simulink model "Quadcopter_model_refined"  (R2022b)
settings: Solver=VariableStepAuto  StartTime=0.0  StopTime=10.0  RelTol=1e-3
undefined symbols (not defined in the file): Cm, Ct, g, initState, Ir, Ixx, Iyy, Izz, Length, mass
libraries: sharedtransform x4, simulink_extras x2, shared6dof x1, aerolibutil x1
settings Model: Creator=Bw Jiang  LastModifiedBy=Bw Jiang

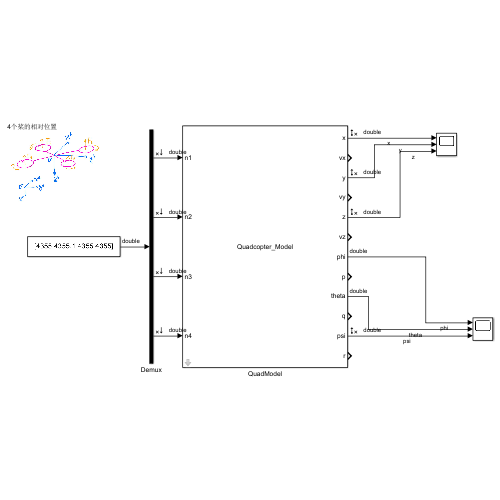
[thumbnail: Simulink's stored preview of the top-level diagram]
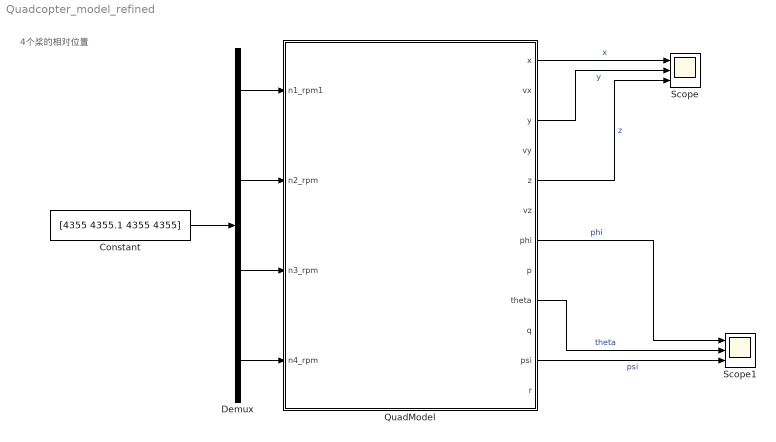
== system Quadcopter_model_refined ==
  note: 4个桨的相对位置
  Constant : Constant  Value=[4355 4355.1 4355 4355]
  Demux : Demux
  QuadModel : Subsystem  mask{g=g, mass=mass, I_xx=Ixx, I_yy=Iyy, I_zz=Izz, I_r=Ir, L=Length, C_M=Cm, C_T=Ct}
      mask prompts: g "Gravity"; I_xx "Inertia_xx"; I_yy "Inertia_yy"; I_zz "Inertia_zz"; I_r "Inertia_per_rotor"; L "Length"
      mask DialogControl ParameterGroupVar Prompt: 参数
      mask Display:
      | disp('Quadcopter_Model');
      | 
      | port_label('input', 1, 'n1');
      | port_label('input', 2, 'n2');
      | port_label('input', 3, 'n3');
      | port_label('input', 4, 'n4');
      | 
      | port_label('output', 1, 'x');
      | port_label('output', 2, 'vx');
      | port_label('output', 3, 'y');
      | port_label('output', 4, 'vy');
      | port_label('output', 5, 'z');
      | port_label('output', 6, 'vz');
      | port_label('output', 7, 'phi');
      | port_label('output', 8, 'p');
      | port_label('output', 9, 'theta');
      | port_label('output', 10, 'q');
      | port_label('output', 11, 'psi');
      | port_label('output', 12, 'r');
  Scope : Scope  NumInputPorts=3
  Scope1 : Scope  NumInputPorts=3
  wires:
  Constant/1 -> Demux/1
  Demux/4 -> QuadModel/4(n4_rpm)
  Demux/1 -> QuadModel/1(n1_rpm1)
  Demux/3 -> QuadModel/3(n3_rpm)
  Demux/2 -> QuadModel/2(n2_rpm)
  QuadModel/1(x) -> Scope/1  "x"
  QuadModel/3(y) -> Scope/2  "y"
  QuadModel/5(z) -> Scope/3  "z"
  QuadModel/11(psi) -> Scope1/3  "psi"
  QuadModel/7(phi) -> Scope1/1  "phi"
  QuadModel/9(theta) -> Scope1/2  "theta"

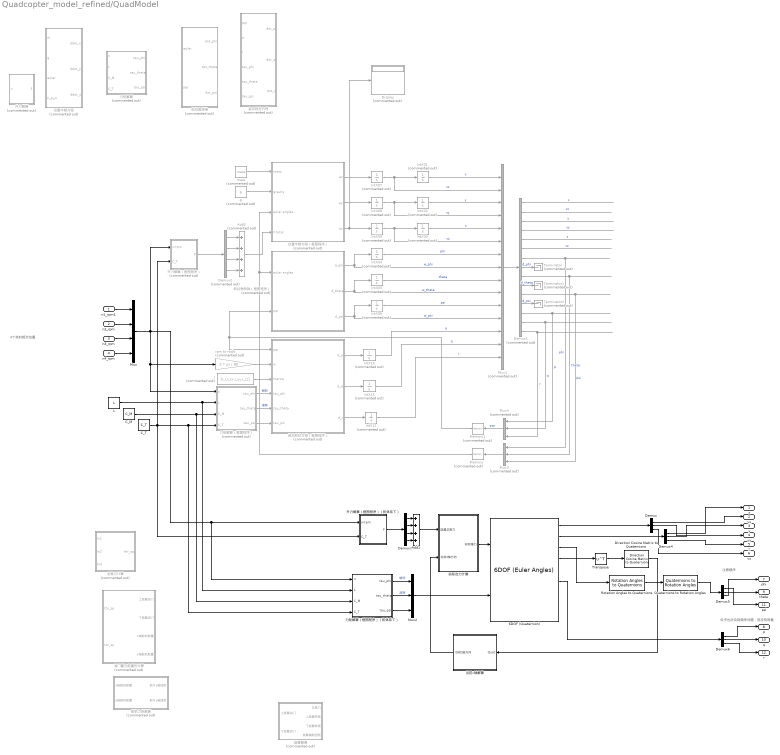
== system Quadcopter_model_refined/QuadModel ==
  note: 似乎也涉及到顺序问题，但没有用着
  note: 注意顺序
  note: 4个桨的相对位置
  n1_rpm1 : Inport
  n2_rpm : Inport  Port=2
  n3_rpm : Inport  Port=3
  n4_rpm : Inport  Port=4
  6DOF (Quaternion) : shared6dof/6DOF (Euler Angles)  units=Metric (MKS)  mtype=Fixed  rep=Euler Angles  xme_0=[initState.x, initState.y, initState.z]  Vm_0=[initState.vx, initState.vy, initState.vz]  eul_0=[initState.phi, initState.theta, initState.psi]  pm_0=[initState.p, initState.q, initState.r]  mass_0=mass  mass_e=0.5  mass_f=2.0  inertia=[Ixx, 0, 0; 0, Iyy, 0; 0, 0, Izz]  inertia_e=eye(3)  inertia_f=2*eye(3)  k_quat=Vehicle.SixDOF.quatGain  vre_flag=on  abi_flag=on  aMode=aMode  xme_statename=''  Vm_statename=''  eul_statename=''  quat_statename=''  pm_statename=''  mass_statename=''
  Add1 : Sum  Inputs=++++
  Add2 : Sum  Commented=on  Inputs=++++
  C_M : Constant  Value=C_M
  C_T : Constant  Value=C_T
  Demux{,4..6} (4 alike) : Demux  Outputs=3
  Demux1 : Demux  Commented=on  Outputs=15
  Demux2 : Demux  Commented=on
  Demux3 : Demux
  Direction Cosine Matrix to Quaternions : sharedtransform/Direction Cosine Matrix  to Quaternions  aMode=0  action=None  tolerance=eps(2)
  Display : Display  Commented=on
  I : Constant  Commented=on  Value=[I_r,I_xx,I_yy,I_zz]
  IntX01 : Integrator  Commented=on
  IntX02 : Integrator  Commented=on
  IntX03 : Integrator  Commented=on
  IntX04 : Integrator  Commented=on
  IntX05 : Integrator  Commented=on
  IntX06 : Integrator  Commented=on
  IntX07 : Integrator  Commented=on
  IntX08 : Integrator  Commented=on
  IntX09 : Integrator  Commented=on
  IntX10 : Integrator  Commented=on
  IntX11 : Integrator  Commented=on
  IntX12 : Integrator  Commented=on
  L : Constant  Value=L
  Memory : Memory  Commented=on  InheritSampleTime=on
  Memory1 : Memory  Commented=on  InheritSampleTime=on
  Mux : Mux
  Mux1 : Mux  Commented=on  Inputs=15
  Mux2 : Mux  Inputs=3
  Mux3 : Mux  Commented=on  Inputs=3
  Mux4 : Mux  Commented=on  Inputs=3
  Quaternions to Rotation Angles : sharedtransform/Quaternions to Rotation Angles  rotationOrder=XYZ  aMode=aMode
  Rotation Angles to Quaternions : sharedtransform/Rotation Angles to Quaternions  rotationOrder=ZYX  aMode=aMode
  Terminator : Terminator  Commented=on
  Terminator1 : Terminator  Commented=on
  Terminator2 : Terminator  Commented=on
  Transpose : Math  Operator=transpose
  g : Constant  Commented=on  Value=g
  mass : Constant  Commented=on  Value=mass
  rpm to rad/s : Gain  Commented=on  Gain=2 * pi / 60
  位置牛顿方程 : MATLAB Function  Commented=on  TreatAsAtomicUnit=on
  位置牛顿方程（框图程序） : Subsystem  Commented=on
  力矩解算 : MATLAB Function  Commented=on  TreatAsAtomicUnit=on
  力矩解算（框图程序） : Subsystem  Commented=on
  力矩解算（框图程序）（机体系下） : Subsystem
  升力解算 : MATLAB Function  Commented=on  TreatAsAtomicUnit=on
  升力解算（框图程序） : Subsystem  Commented=on
  升力解算（框图程序）（机体系下） : Subsystem
  姿态欧拉方程 : MATLAB Function  Commented=on  TreatAsAtomicUnit=on
  姿态欧拉方程（框图程序） : Subsystem  Commented=on
  实际合力计算 : Subsystem
  当前z轴解算 : Subsystem
  总推力计算 : Subsystem  Commented=on
  旋翼解算 : Subsystem  Commented=on
  欧拉角转换 : MATLAB Function  Commented=on  TreatAsAtomicUnit=on
  欧拉角转换（框图程序） : Subsystem  Commented=on
  油门量与舵量的计算 : Subsystem  Commented=on
  舵机力矩解算 : Subsystem  Commented=on
  x : Outport
  vx : Outport  Port=2
  y : Outport  Port=3
  vy : Outport  Port=4
  z : Outport  Port=5
  vz : Outport  Port=6
  phi : Outport  Port=7
  p : Outport  Port=8
  theta : Outport  Port=9
  q : Outport  Port=10
  psi : Outport  Port=11
  r : Outport  Port=12
  wires:
  Demux1/15 -> Mux4/3  "r"
  Demux1/13 -> Mux4/1  "p"
  Mux4/1 -> Memory1/1  "pqr"
  Demux1/9 -> Mux3/2  "theta"
  Demux1/1 -> ?  "x"
  Demux1/2 -> ?  "vx"
  Demux1/11 -> Mux3/3  "psi"
  Demux1/4 -> ?  "vy"
  Demux1/3 -> ?  "y"
  Demux1/5 -> ?  "z"
  Mux1/1 -> Demux1/1
  Demux1/6 -> ?  "vz"
  Demux1/7 -> Mux3/1  "phi"
  Mux3/1 -> Memory/1
  Demux1/14 -> Mux4/2  "q"
  Demux1/8 -> Terminator/1  "d_phi"
  Demux1/10 -> Terminator1/1  "d_theta"
  Demux1/12 -> Terminator2/1  "d_psi"
  n1_rpm1/1 -> Mux/1
  n2_rpm/1 -> Mux/2
  n4_rpm/1 -> Mux/4
  n3_rpm/1 -> Mux/3
  欧拉角转换（框图程序）/2(d_theta) -> IntX05/1, Mux1/10  "w_theta"
  欧拉角转换（框图程序）/3(d_psi) -> IntX06/1, Mux1/12  "w_psi"
  欧拉角转换（框图程序）/1(d_phi) -> IntX04/1, Mux1/8  "w_phi"
  力矩解算（框图程序）/3(tau_psi) -> 姿态欧拉方程（框图程序）/6(tau_psi)
  力矩解算（框图程序）/2(tau_theta) -> 姿态欧拉方程（框图程序）/5(tau_theta)  "滚转"
  姿态欧拉方程（框图程序）/2(d_q) -> IntX11/1
  姿态欧拉方程（框图程序）/3(d_r) -> IntX12/1
  mass/1 -> 位置牛顿方程（框图程序）/1(mass)
  Add2/1 -> 位置牛顿方程（框图程序）/4(F total)
  g/1 -> 位置牛顿方程（框图程序）/2(gravity)
  位置牛顿方程（框图程序）/3(az) -> Display/1, IntX09/1
  位置牛顿方程（框图程序）/2(ay) -> IntX08/1
  IntX05/1 -> Mux1/9  "theta"
  力矩解算（框图程序）/1(tau_phi) -> 姿态欧拉方程（框图程序）/4(tau_phi)  "俯仰"
  IntX07/1 -> IntX01/1, Mux1/2  "vx"
  IntX02/1 -> Mux1/3  "y"
  Demux2/3 -> Add2/3
  IntX12/1 -> Mux1/15  "r"
  rpm to rad/s/1 -> 姿态欧拉方程（框图程序）/2(w)
  IntX06/1 -> Mux1/11  "psi"
  IntX08/1 -> Mux1/4, IntX02/1  "vy"
  Mux/1 -> 力矩解算（框图程序）（机体系下）/1(n), 升力解算（框图程序）（机体系下）/1(n/rpm), 力矩解算（框图程序）/1(n), rpm to rad/s/1, 升力解算（框图程序）/1(n/rpm)
  Memory1/1 -> 欧拉角转换（框图程序）/2(pqr), 姿态欧拉方程（框图程序）/1(pqr)
  位置牛顿方程（框图程序）/1(ax) -> IntX07/1
  Demux2/1 -> Add2/1
  IntX01/1 -> Mux1/1  "x"
  IntX11/1 -> Mux1/14  "q"
  姿态欧拉方程（框图程序）/1(d_p) -> IntX10/1
  IntX04/1 -> Mux1/7  "phi"
  Demux2/2 -> Add2/2
  L/1 -> 力矩解算（框图程序）（机体系下）/2(L), 力矩解算（框图程序）/2(L)
  I/1 -> 姿态欧拉方程（框图程序）/3(Inertia)
  C_M/1 -> 力矩解算（框图程序）（机体系下）/3(C_M), 力矩解算（框图程序）/3(C_M)
  升力解算（框图程序）/1(F) -> Demux2/1
  C_T/1 -> 升力解算（框图程序）（机体系下）/2(C_T), 升力解算（框图程序）/2(C_T), 力矩解算（框图程序）（机体系下）/4(C_T), 力矩解算（框图程序）/4(C_T)
  IntX03/1 -> Mux1/5  "z"
  Demux2/4 -> Add2/4
  IntX09/1 -> Mux1/6, IntX03/1  "vz"
  IntX10/1 -> Mux1/13  "p"
  Memory/1 -> 位置牛顿方程（框图程序）/3(eular angles), 欧拉角转换（框图程序）/1(eular angles)
  实际合力计算/1(实际推力) -> 6DOF (Quaternion)/1
  6DOF (Quaternion)/4 -> Transpose/1
  Transpose/1 -> Direction Cosine Matrix to Quaternions/1
  Direction Cosine Matrix to Quaternions/1 -> 当前z轴解算/1(Quat)
  当前z轴解算/1(当前z轴方向) -> 实际合力计算/2(当前z轴方向)
  Demux3/1 -> Add1/1
  Demux3/4 -> Add1/4
  升力解算（框图程序）（机体系下）/1(F) -> Demux3/1
  Demux3/2 -> Add1/2
  Demux3/3 -> Add1/3
  Add1/1 -> 实际合力计算/1(旋翼总推力)
  力矩解算（框图程序）（机体系下）/3(tau_psi) -> Mux2/3
  力矩解算（框图程序）（机体系下）/2(tau_theta) -> Mux2/2  "滚转"
  力矩解算（框图程序）（机体系下）/1(tau_phi) -> Mux2/1  "俯仰"
  Mux2/1 -> 6DOF (Quaternion)/2
  6DOF (Quaternion)/1 -> Demux/1
  6DOF (Quaternion)/2 -> Demux4/1
  Demux4/1 -> x/1
  Demux4/2 -> y/1
  Demux4/3 -> z/1
  Demux/1 -> vx/1
  Demux/2 -> vy/1
  Demux/3 -> vz/1
  6DOF (Quaternion)/3 -> Rotation Angles to Quaternions/1
  Rotation Angles to Quaternions/1 -> Quaternions to Rotation Angles/1
  Quaternions to Rotation Angles/1 -> Demux5/1
  Demux5/1 -> psi/1
  Demux5/2 -> theta/1
  Demux5/3 -> phi/1
  6DOF (Quaternion)/6 -> Demux6/1
  Demux6/1 -> p/1
  Demux6/2 -> q/1
  Demux6/3 -> r/1

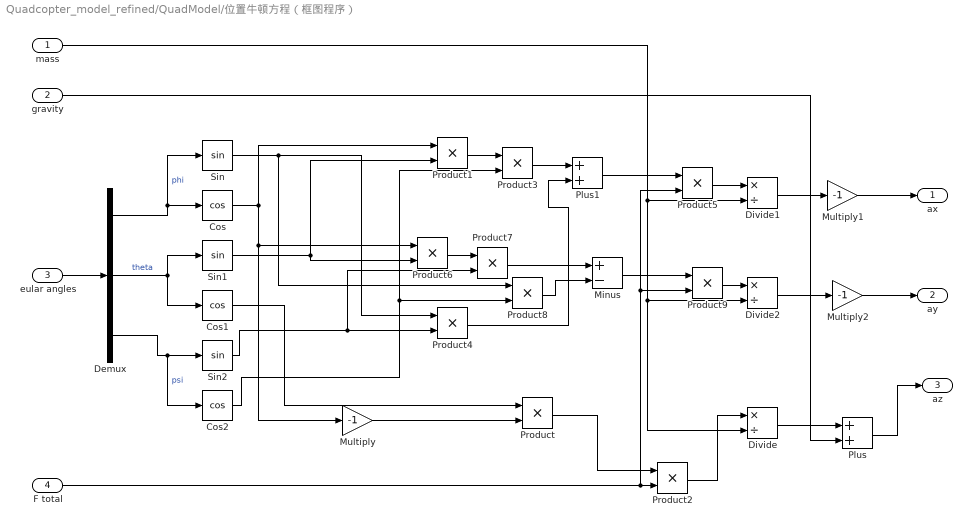
== system Quadcopter_model_refined/QuadModel/位置牛顿方程（框图程序） ==
  mass : Inport
  gravity : Inport  Port=2
  eular angles : Inport  Port=3
  F total : Inport  Port=4
  Cos : Trigonometry  Operator=cos
  Cos1 : Trigonometry  Operator=cos
  Cos2 : Trigonometry  Operator=cos
  Demux : Demux  Outputs=3
  Divide : Product  Inputs=*/
  Divide1 : Product  Inputs=*/
  Divide2 : Product  Inputs=*/
  Minus : Sum  Inputs=+-
  Multiply : Gain  Gain=-1
  Multiply1 : Gain  Gain=-1
  Multiply2 : Gain  Gain=-1
  Plus : Sum
  Plus1 : Sum
  Product{,1..9} (10 alike) : Product
  Sin : Trigonometry
  Sin1 : Trigonometry
  Sin2 : Trigonometry
  ax : Outport
  ay : Outport  Port=2
  az : Outport  Port=3
  wires:
  eular angles/1 -> Demux/1
  Demux/1 -> Sin/1, Cos/1  "phi"
  Demux/2 -> Sin1/1, Cos1/1  "theta"
  Demux/3 -> Cos2/1, Sin2/1  "psi"
  Cos/1 -> Product6/1, Multiply/1, Product1/1
  Multiply/1 -> Product/2
  Cos1/1 -> Product/1
  F total/1 -> Product5/2, Product9/2, Product2/2
  Product/1 -> Product2/1
  Product2/1 -> Divide/1
  mass/1 -> Divide2/2, Divide/2, Divide1/2
  Divide/1 -> Plus/1
  gravity/1 -> Plus/2
  Plus/1 -> az/1
  Sin1/1 -> Product1/2, Product6/2
  Product1/1 -> Product3/1
  Cos2/1 -> Product8/2, Product3/2
  Product3/1 -> Plus1/1
  Sin/1 -> Product8/1, Product4/1
  Sin2/1 -> Product7/2, Product4/2
  Product4/1 -> Plus1/2
  Plus1/1 -> Product5/1
  Product5/1 -> Divide1/1
  Divide1/1 -> Multiply1/1
  Multiply1/1 -> ax/1
  Product6/1 -> Product7/1
  Product7/1 -> Minus/1
  Product8/1 -> Minus/2
  Minus/1 -> Product9/1
  Product9/1 -> Divide2/1
  Multiply2/1 -> ay/1
  Divide2/1 -> Multiply2/1

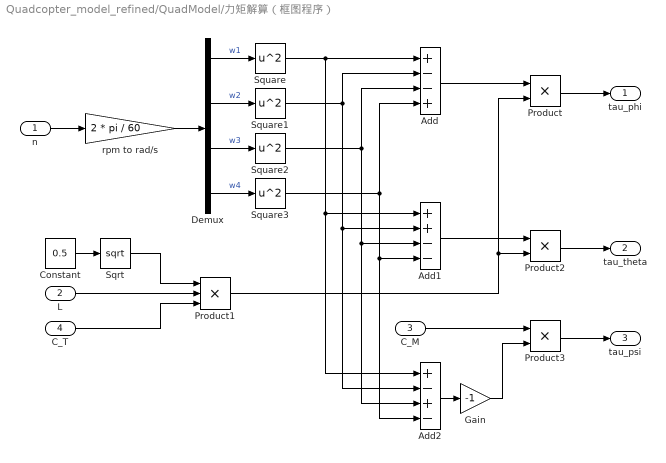
== system Quadcopter_model_refined/QuadModel/力矩解算（框图程序） ==
  n : Inport
  L : Inport  Port=2
  C_M : Inport  Port=3
  C_T : Inport  Port=4
  Add : Sum  Inputs=+--+
  Add1 : Sum  Inputs=++--
  Add2 : Sum  Inputs=+-+-
  Constant : Constant  Value=0.5
  Demux : Demux
  Gain : Gain  Gain=-1
  Product : Product
  Product1 : Product  Inputs=3
  Product2 : Product
  Product3 : Product
  Sqrt : Sqrt
  Square{,1..3} (4 alike) : Math  Operator=square
  rpm to rad/s : Gain  Gain=2 * pi / 60
  tau_phi : Outport
  tau_theta : Outport  Port=2
  tau_psi : Outport  Port=3
  wires:
  rpm to rad/s/1 -> Demux/1
  n/1 -> rpm to rad/s/1
  Demux/1 -> Square/1  "w1"
  Demux/2 -> Square1/1  "w2"
  Demux/3 -> Square2/1  "w3"
  Demux/4 -> Square3/1  "w4"
  Square/1 -> Add1/1, Add2/1, Add/1
  Square1/1 -> Add1/2, Add2/2, Add/2
  Square2/1 -> Add2/3, Add1/3, Add/3
  Square3/1 -> Add2/4, Add1/4, Add/4
  Add/1 -> Product/1
  L/1 -> Product1/2
  C_T/1 -> Product1/3
  Constant/1 -> Sqrt/1
  Sqrt/1 -> Product1/1
  Product1/1 -> Product/2, Product2/2
  Product/1 -> tau_phi/1
  Add1/1 -> Product2/1
  Product2/1 -> tau_theta/1
  Add2/1 -> Gain/1
  C_M/1 -> Product3/1
  Product3/1 -> tau_psi/1
  Gain/1 -> Product3/2

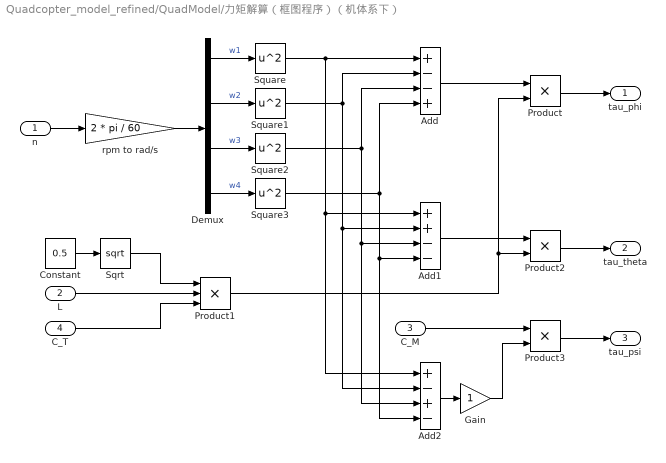
== system Quadcopter_model_refined/QuadModel/力矩解算（框图程序）（机体系下） ==
  n : Inport
  L : Inport  Port=2
  C_M : Inport  Port=3
  C_T : Inport  Port=4
  Add : Sum  Inputs=+--+
  Add1 : Sum  Inputs=++--
  Add2 : Sum  Inputs=+-+-
  Constant : Constant  Value=0.5
  Demux : Demux
  Gain : Gain
  Product : Product
  Product1 : Product  Inputs=3
  Product2 : Product
  Product3 : Product
  Sqrt : Sqrt
  Square{,1..3} (4 alike) : Math  Operator=square
  rpm to rad/s : Gain  Gain=2 * pi / 60
  tau_phi : Outport
  tau_theta : Outport  Port=2
  tau_psi : Outport  Port=3
  wires:
  rpm to rad/s/1 -> Demux/1
  n/1 -> rpm to rad/s/1
  Demux/1 -> Square/1  "w1"
  Demux/2 -> Square1/1  "w2"
  Demux/3 -> Square2/1  "w3"
  Demux/4 -> Square3/1  "w4"
  Square/1 -> Add1/1, Add2/1, Add/1
  Square1/1 -> Add1/2, Add2/2, Add/2
  Square2/1 -> Add2/3, Add1/3, Add/3
  Square3/1 -> Add2/4, Add1/4, Add/4
  Add/1 -> Product/1
  L/1 -> Product1/2
  C_T/1 -> Product1/3
  Constant/1 -> Sqrt/1
  Sqrt/1 -> Product1/1
  Product1/1 -> Product/2, Product2/2
  Product/1 -> tau_phi/1
  Add1/1 -> Product2/1
  Product2/1 -> tau_theta/1
  Add2/1 -> Gain/1
  C_M/1 -> Product3/1
  Product3/1 -> tau_psi/1
  Gain/1 -> Product3/2

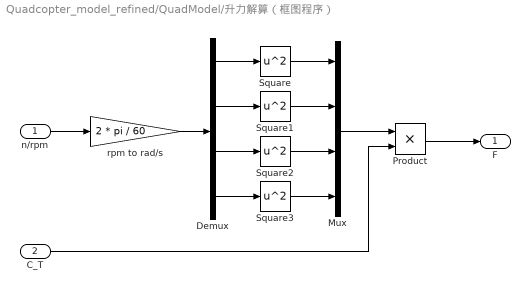
== system Quadcopter_model_refined/QuadModel/升力解算（框图程序） ==
  n/rpm : Inport
  C_T : Inport  Port=2
  Demux : Demux
  Mux : Mux
  Product : Product
  Square{,1..3} (4 alike) : Math  Operator=square
  rpm to rad/s : Gain  Gain=2 * pi / 60
  F : Outport
  wires:
  n/rpm/1 -> rpm to rad/s/1
  rpm to rad/s/1 -> Demux/1
  Demux/1 -> Square/1
  Demux/2 -> Square1/1
  Demux/3 -> Square2/1
  Demux/4 -> Square3/1
  Square3/1 -> Mux/4
  Square2/1 -> Mux/3
  Square1/1 -> Mux/2
  Square/1 -> Mux/1
  Mux/1 -> Product/1
  C_T/1 -> Product/2
  Product/1 -> F/1

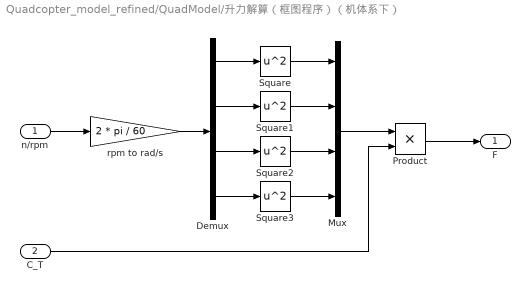
== system Quadcopter_model_refined/QuadModel/升力解算（框图程序）（机体系下） ==
  n/rpm : Inport
  C_T : Inport  Port=2
  Demux : Demux
  Mux : Mux
  Product : Product
  Square{,1..3} (4 alike) : Math  Operator=square
  rpm to rad/s : Gain  Gain=2 * pi / 60
  F : Outport
  wires:
  n/rpm/1 -> rpm to rad/s/1
  rpm to rad/s/1 -> Demux/1
  Demux/1 -> Square/1
  Demux/2 -> Square1/1
  Demux/3 -> Square2/1
  Demux/4 -> Square3/1
  Square3/1 -> Mux/4
  Square2/1 -> Mux/3
  Square1/1 -> Mux/2
  Square/1 -> Mux/1
  Mux/1 -> Product/1
  C_T/1 -> Product/2
  Product/1 -> F/1

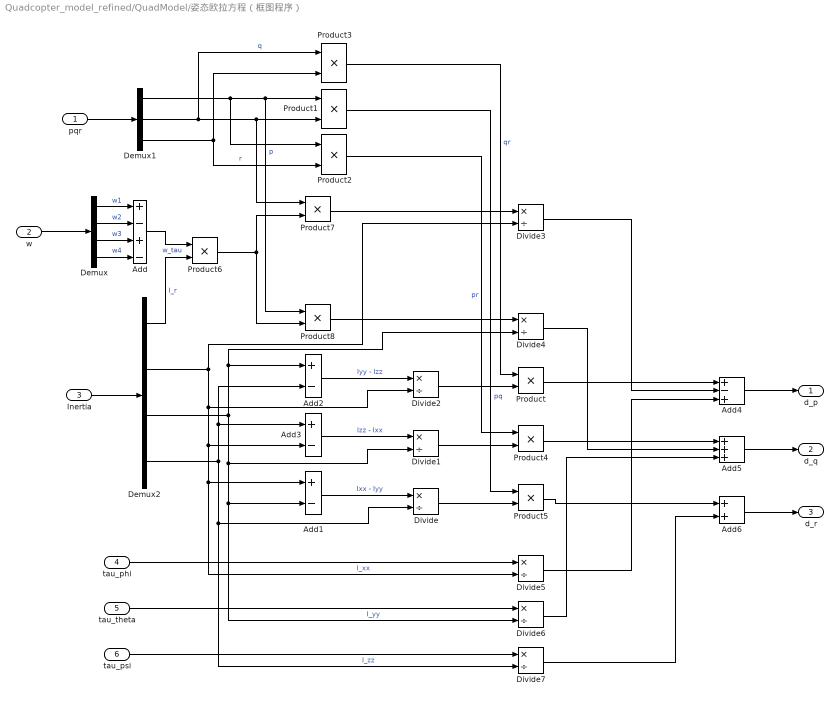
== system Quadcopter_model_refined/QuadModel/姿态欧拉方程（框图程序） ==
  pqr : Inport
  w : Inport  Port=2
  Inertia : Inport  Port=3
  tau_phi : Inport  Port=4
  tau_theta : Inport  Port=5
  tau_psi : Inport  Port=6
  Add : Sum  Inputs=+-+-
  Add1 : Sum  Inputs=+-
  Add2 : Sum  Inputs=+-
  Add3 : Sum  Inputs=+-
  Add4 : Sum  Inputs=+-+
  Add5 : Sum  Inputs=+++
  Add6 : Sum
  Demux : Demux
  Demux1 : Demux  Outputs=3
  Demux2 : Demux
  Divide{,1..7} (8 alike) : Product  Inputs=*/
  Product{,1..8} (9 alike) : Product
  d_p : Outport
  d_q : Outport  Port=2
  d_r : Outport  Port=3
  wires:
  w/1 -> Demux/1
  pqr/1 -> Demux1/1
  Inertia/1 -> Demux2/1
  Demux/1 -> Add/1  "w1"
  Demux/2 -> Add/2  "w2"
  Demux/3 -> Add/3  "w3"
  Demux/4 -> Add/4  "w4"
  Demux2/2 -> Add3/2, Add1/1, Divide5/2, Divide2/2, Divide3/2  "I_xx"
  Demux2/3 -> Divide4/2, Add2/1, Divide1/2, Divide6/2, Add1/2  "I_yy"
  Demux2/4 -> Add2/2, Add3/1, Divide7/2, Divide/2  "I_zz"
  Add1/1 -> Divide/1  "Ixx - Iyy"
  Add3/1 -> Divide1/1  "Izz - Ixx"
  Add2/1 -> Divide2/1  "Iyy - Izz"
  Divide2/1 -> Product/2
  Demux1/2 -> Product3/1, Product1/2, Product7/1  "q"
  Demux1/1 -> Product2/1, Product1/1, Product8/1  "p"
  Demux1/3 -> Product2/2, Product3/2  "r"
  Divide/1 -> Product5/2
  Divide1/1 -> Product4/2
  Product3/1 -> Product/1  "qr"
  Product1/1 -> Product5/1  "pq"
  Product2/1 -> Product4/1  "pr"
  Add/1 -> Product6/1  "w_tau"
  Demux2/1 -> Product6/2  "I_r"
  Product6/1 -> Product8/2, Product7/2
  Product7/1 -> Divide3/1
  Product8/1 -> Divide4/1
  tau_phi/1 -> Divide5/1
  tau_theta/1 -> Divide6/1
  tau_psi/1 -> Divide7/1
  Product/1 -> Add4/1
  Divide3/1 -> Add4/2
  Divide5/1 -> Add4/3
  Product4/1 -> Add5/1
  Divide4/1 -> Add5/2
  Divide6/1 -> Add5/3
  Add4/1 -> d_p/1
  Add5/1 -> d_q/1
  Product5/1 -> Add6/1
  Divide7/1 -> Add6/2
  Add6/1 -> d_r/1

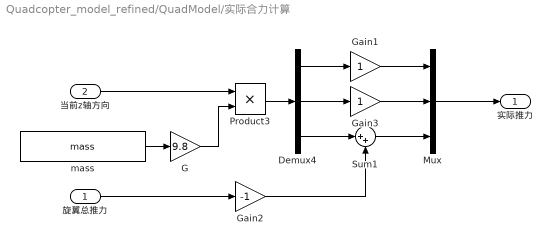
== system Quadcopter_model_refined/QuadModel/实际合力计算 ==
  旋翼总推力 : Inport
  当前z轴方向 : Inport  Port=2
  Demux4 : Demux  Outputs=3
  G : Gain  Gain=9.8
  Gain1 : Gain
  Gain2 : Gain  Gain=-1
  Gain3 : Gain
  Mux : Mux  Inputs=3
  Product3 : Product
  Sum1 : Sum  Inputs=|++
  mass : Constant  Value=mass
  实际推力 : Outport
  wires:
  Demux4/1 -> Gain1/1
  当前z轴方向/1 -> Product3/1
  G/1 -> Product3/2
  Sum1/1 -> Mux/3
  Demux4/2 -> Gain3/1
  mass/1 -> G/1
  Product3/1 -> Demux4/1
  Mux/1 -> 实际推力/1
  旋翼总推力/1 -> Gain2/1
  Gain1/1 -> Mux/1
  Gain3/1 -> Mux/2
  Demux4/3 -> Sum1/1
  Gain2/1 -> Sum1/2

== system Quadcopter_model_refined/QuadModel/当前z轴解算 ==
  Quat : Inport
  Demux5 : Demux  Outputs=3
  Display : Display
  Display1 : Display
  Quaternion Inverse : aerolibutil/Quaternion Inverse
  Quaternions to Direction Cosine Matrix : sharedtransform/Quaternions to  Direction Cosine Matrix  aMode=aMode
  Reshape2 : Reshape  OutputDimensionality=Row vector (2-D)
  ez : Scope
  一列一列地读取形成向量 : Reshape  OutputDimensionality=Column vector (2-D)
  当前z轴方向 : Outport
  wires:
  Quat/1 -> Quaternion Inverse/1
  Demux5/3 -> Reshape2/1
  Reshape2/1 -> 当前z轴方向/1, ez/1
  Quaternions to Direction Cosine Matrix/1 -> Display/1, 一列一列地读取形成向量/1
  一列一列地读取形成向量/1 -> Display1/1, Demux5/1
  Quaternion Inverse/1 -> Quaternions to Direction Cosine Matrix/1

== system Quadcopter_model_refined/QuadModel/总推力计算 ==
  In1 : Inport
  In2 : Inport  Port=2
  In3 : Inport  Port=3
  Sqrt : Sqrt
  Square : Math  Operator=square
  Square1 : Math  Operator=square
  Square2 : Math  Operator=square
  Sum1 : Sum  Inputs=+++
  thr_sp : Outport
  wires:
  Sum1/1 -> Sqrt/1
  Square1/1 -> Sum1/2
  Square/1 -> Sum1/1
  Square2/1 -> Sum1/3
  Sqrt/1 -> thr_sp/1  "thr_sp"
  In2/1 -> Square1/1
  In3/1 -> Square2/1
  In1/1 -> Square/1

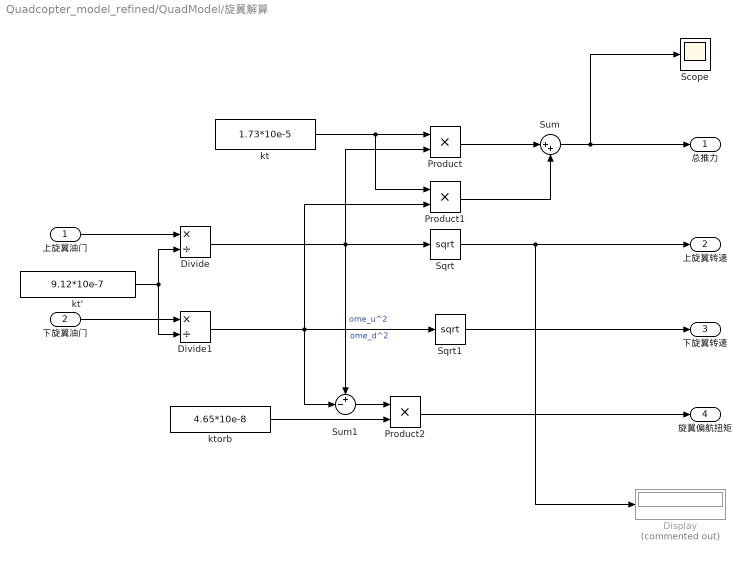
== system Quadcopter_model_refined/QuadModel/旋翼解算 ==
  上旋翼油门 : Inport
  下旋翼油门 : Inport  Port=2
  Display : Display  Commented=on
  Divide : Product  Inputs=*/
  Divide1 : Product  Inputs=*/
  Product : Product
  Product1 : Product
  Product2 : Product
  Scope : Scope
  Sqrt : Sqrt
  Sqrt1 : Sqrt
  Sum : Sum  Inputs=|++
  Sum1 : Sum  Inputs=+-|
  kt : Constant  Value=1.73*10e-5
  kt' : Constant  Value=9.12*10e-7
  ktorb : Constant  Value=4.65*10e-8
  总推力 : Outport
  上旋翼转速 : Outport  Port=2
  下旋翼转速 : Outport  Port=3
  旋翼偏航扭矩 : Outport  Port=4
  wires:
  上旋翼油门/1 -> Divide/1
  kt'/1 -> Divide1/2, Divide/2
  下旋翼油门/1 -> Divide1/1
  Divide/1 -> Sqrt/1, Product/2, Sum1/1  "ome_u^2"
  Sqrt/1 -> Display/1, 上旋翼转速/1
  Divide1/1 -> Sqrt1/1, Product1/2, Sum1/2  "ome_d^2"
  Sqrt1/1 -> 下旋翼转速/1
  kt/1 -> Product/1, Product1/1
  Product/1 -> Sum/1
  Sum/1 -> Scope/1, 总推力/1
  Product1/1 -> Sum/2
  Sum1/1 -> Product2/1
  ktorb/1 -> Product2/2
  Product2/1 -> 旋翼偏航扭矩/1

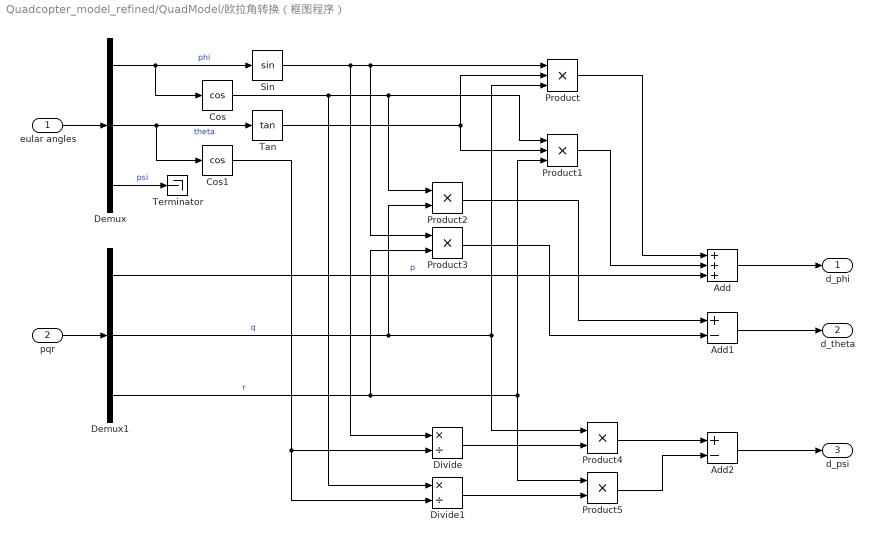
== system Quadcopter_model_refined/QuadModel/欧拉角转换（框图程序） ==
  eular angles : Inport
  pqr : Inport  Port=2
  Add : Sum  Inputs=+++
  Add1 : Sum  Inputs=+-
  Add2 : Sum  Inputs=+-
  Cos : Trigonometry  Operator=cos
  Cos1 : Trigonometry  Operator=cos
  Demux : Demux  Outputs=3
  Demux1 : Demux  Outputs=3
  Divide : Product  Inputs=*/
  Divide1 : Product  Inputs=*/
  Product : Product  Inputs=3
  Product1 : Product  Inputs=3
  Product{2..5} (4 alike) : Product
  Sin : Trigonometry
  Tan : Trigonometry  Operator=tan
  Terminator : Terminator
  d_phi : Outport
  d_theta : Outport  Port=2
  d_psi : Outport  Port=3
  wires:
  eular angles/1 -> Demux/1
  pqr/1 -> Demux1/1
  Demux1/1 -> Add/3  "p"
  Add/1 -> d_phi/1
  Add1/1 -> d_theta/1
  Add2/1 -> d_psi/1
  Demux/1 -> Sin/1, Cos/1  "phi"
  Demux/2 -> Cos1/1, Tan/1  "theta"
  Demux/3 -> Terminator/1  "psi"
  Demux1/2 -> Product2/2, Product4/1, Product/3  "q"
  Sin/1 -> Divide/1, Product3/1, Product/1
  Tan/1 -> Product1/2, Product/2
  Cos/1 -> Divide1/1, Product2/1, Product1/1
  Demux1/3 -> Product3/2, Product1/3, Product5/1  "r"
  Product/1 -> Add/1
  Product1/1 -> Add/2
  Product2/1 -> Add1/1
  Product3/1 -> Add1/2
  Cos1/1 -> Divide1/2, Divide/2
  Divide/1 -> Product4/2
  Product4/1 -> Add2/1
  Divide1/1 -> Product5/2
  Product5/1 -> Add2/2

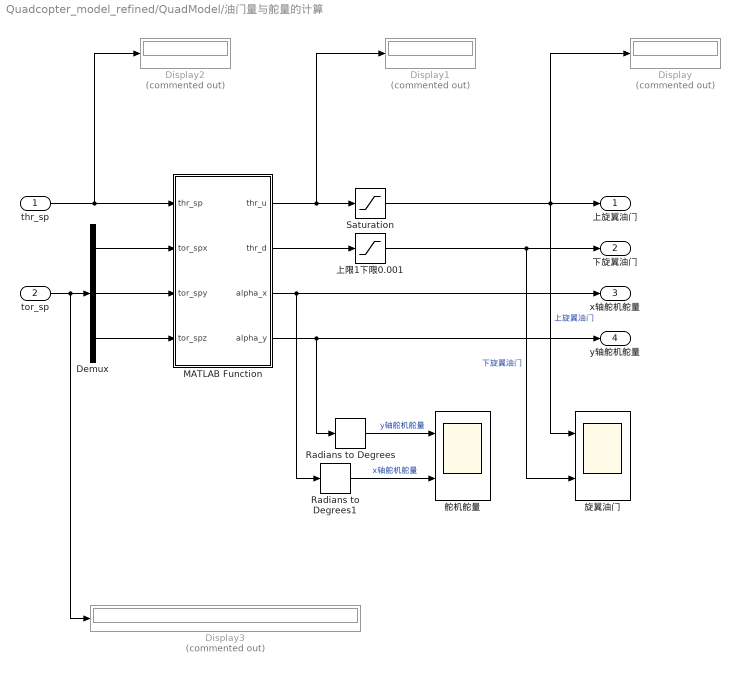
== system Quadcopter_model_refined/QuadModel/油门量与舵量的计算 ==
  thr_sp : Inport
  tor_sp : Inport  Port=2
  Demux : Demux  Outputs=3
  Display{,1..3} (4 alike) : Display  Commented=on
  MATLAB Function : MATLAB Function  TreatAsAtomicUnit=on
  Radians to Degrees : simulink_extras/Transformations/Radians to Degrees
  Radians to Degrees1 : simulink_extras/Transformations/Radians to Degrees
  Saturation : Saturate  UpperLimit=1  LowerLimit=0.001
  上限1下限0.001 : Saturate  UpperLimit=1  LowerLimit=0.001
  旋翼油门 : Scope  NumInputPorts=2
  舵机舵量 : Scope  NumInputPorts=2
  上旋翼油门 : Outport
  下旋翼油门 : Outport  Port=2
  x轴舵机舵量 : Outport  Port=3
  y轴舵机舵量 : Outport  Port=4
  wires:
  MATLAB Function/1(thr_u) -> Display1/1, Saturation/1
  Radians to Degrees/1 -> 舵机舵量/1  "y轴舵机舵量"
  MATLAB Function/3(alpha_x) -> x轴舵机舵量/1, Radians to Degrees1/1
  Radians to Degrees1/1 -> 舵机舵量/2  "x轴舵机舵量"
  Saturation/1 -> 旋翼油门/1, Display/1, 上旋翼油门/1  "上旋翼油门"
  上限1下限0.001/1 -> 下旋翼油门/1, 旋翼油门/2  "下旋翼油门"
  MATLAB Function/4(alpha_y) -> y轴舵机舵量/1, Radians to Degrees/1
  Demux/2 -> MATLAB Function/3(tor_spy)
  thr_sp/1 -> Display2/1, MATLAB Function/1(thr_sp)
  Demux/3 -> MATLAB Function/4(tor_spz)
  MATLAB Function/2(thr_d) -> 上限1下限0.001/1
  Demux/1 -> MATLAB Function/2(tor_spx)
  tor_sp/1 -> Display3/1, Demux/1

== system Quadcopter_model_refined/QuadModel/舵机力矩解算 ==
  x轴舵机舵量 : Inport
  y轴舵机舵量 : Inport  Port=2
  MATLAB Function : MATLAB Function  TreatAsAtomicUnit=on
  舵片x轴扭矩 : Outport
  舵片y轴扭矩 : Outport  Port=2
  wires:
  x轴舵机舵量/1 -> MATLAB Function/1(ax)
  y轴舵机舵量/1 -> MATLAB Function/2(ay)
  MATLAB Function/1(tx) -> 舵片x轴扭矩/1
  MATLAB Function/2(ty) -> 舵片y轴扭矩/1

== matlab function Quadcopter_model_refined/QuadModel/油门量与舵量的计算/MATLAB Function ==
  data: thr_sp input; thr_u output; tor_spx input; tor_spy input; tor_spz input; thr_d output; alpha_x output; alpha_y output
function [thr_u,thr_d,alpha_x,alpha_y] = fcn(thr_sp,tor_spx,tor_spy,tor_spz)
%A为伪控制量到双桨转速、两组舵机舵量（弧度）的控制分配矩阵
A = [1,0.098,0,0;1,-0.098,0,0;0,0,1.047,0;0,0,0,1.047];
B= A*[thr_sp;tor_spz;tor_spx;tor_spy];
thr_u = B(1);
thr_d = B(2);
alpha_x = B(3);
alpha_y = B(4);

== matlab function Quadcopter_model_refined/QuadModel/舵机力矩解算/MATLAB Function ==
  data: ax input; tx output; ay input; ty output
function [tx, ty] = fcn(ax, ay)

if ax > 0
    tx = 2 * 1.24 * 20 * (0.05 * 0.1) * sin(ax)^2 * 2 * 20 * (0.5 * 0.05 + 0.1 * cos(ax));
else
    tx = -2 * 1.24 * 20 * (0.05 * 0.1) * sin(ax)^2 * 2 * 20 * (0.5 * 0.05 + 0.1 * cos(ax));
end

if ay > 0
    ty = 2 * 1.24 * 20 * (0.05 * 0.1) * sin(ay)^2 * 2 * 20 * (0.5 * 0.05 + 0.1 * cos(ay));
else
    ty = -2 * 1.24 * 20 * (0.05 * 0.1) * sin(ay)^2 * 2 * 20 * (0.5 * 0.05 + 0.1 * cos(ay));
end

== matlab function Quadcopter_model_refined/QuadModel/欧拉角转换 ==
  data: euler input; pqr input; dot_phi output; dot_theta output; dot_psi output
function [dot_phi, dot_theta, dot_psi] = fcn(euler, pqr)

% 角加速度的坐标转换，从机体系b到惯性系e

p = pqr(1);
q = pqr(2);
r = pqr(3);

phi =euler(1);
theta = euler(2);
psi = euler(3);

mat = [
    1, tan(theta) * sin(phi), tan(theta) * cos(phi);
    0, cos(phi), -sin(phi);
    0, sin(phi) / cos(theta), cos(phi) / cos(theta)
    ];
body = [p; q; r];
earth = mat * body;

dot_phi = earth(1);
dot_theta = earth(2);
dot_psi = earth(3);

end

== matlab function Quadcopter_model_refined/QuadModel/位置牛顿方程 ==
  data: m input; g input; euler input; ddot_x output; F_sum input; ddot_y output; ddot_z output
function [ddot_x, ddot_y, ddot_z] = fcn(m, g, euler, F_sum)

% F_sum恒正

phi = euler(1);
theta = euler(2);
psi = euler(3);

ddot_x = -(cos(phi) * sin(theta) * cos(psi) + sin(phi) * sin(psi)) * F_sum / m;
ddot_y = -(cos(phi) * sin(theta) * sin(psi) - sin(phi) * cos(psi)) * F_sum / m;
ddot_z = -cos(phi) * cos(theta) * F_sum / m + g;

end

== matlab function Quadcopter_model_refined/QuadModel/力矩解算 ==
  data: n input; L input; tau_phi output; tau_theta output; tau_psi output; C_M input; C_T input
function [tau_phi, tau_theta, tau_psi]= fcn(n, L, C_M, C_T)
%% Input Vars
% n - rpm
% L - m
% C_M - N*m*s^2/rad^2
% C_T - N*s^2/rad^2

%% Output Vars
% tau - N*m

%% Mid Vars
% w - rad/s

%% Code

% C_T = 1.1e-5;
% C_M = 1.0144e-7;

% F1 = F(1);
% F2 = F(2);
% F3 = F(3);
% F4 = F(4);

w1 = n(1) / 60 * 2 * pi;
w2 = n(2) / 60 * 2 * pi;
w3 = n(3) / 60 * 2 * pi;
w4 = n(4) / 60 * 2 * pi;

% I_r = I(1);

% w_tau = w1 + w3 - w2 - w4;

% 横滚
tau_phi = sqrt(2) / 2 * C_T * L * (w1^2 - w2^2 - w3^2 + w4^2); % tau_phi = (F1+F2-F3-F4) * L;
% 俯仰
tau_theta = sqrt(2) / 2 * C_T * L * (w1^2 + w2^2 - w3^2 - w4^2); % tau_theta = (F1-F2-F3+F4) * L;
% 偏航
tau_psi = C_M * (w1^2 - w2^2 + w3^2 - w4^2); % tau_psi = w_tau * I_r;

end

== matlab function Quadcopter_model_refined/QuadModel/升力解算 ==
  data: n input; F output
function F = fcn(n)
%% Input Vars
% n - rpm

%% Output Vars
% F - N

%% Mid Vars
% omega - rad/s

%% Code

% F = n .* n * 2.414e-7 * 2;

omega = n / 60 * 2 * pi;
F = omega .* omega * 1.11e-5;

end

== matlab function Quadcopter_model_refined/QuadModel/姿态欧拉方程 ==
  data: pqr input; dot_p output; w input; I input; dot_q output; dot_r output; tau_phi input; tau_theta input; tau_psi input
function [dot_p, dot_q, dot_r] = fcn(pqr, w, I, tau_phi, tau_theta, tau_psi)

w1 = w(1);
w2 = w(2);
w3 = w(3);
w4 = w(4);

p = pqr(1);
q = pqr(2);
r = pqr(3);

I_r = I(1);
I_xx = I(2);
I_yy = I(3);
I_zz = I(4);

w_tau = w1 - w2 + w3 - w4;

dot_p = (I_yy - I_zz) / I_xx * q * r - I_r * q / I_xx * w_tau + tau_phi / I_xx;
dot_q = (I_zz - I_xx) / I_yy * p * r + I_r * p / I_yy * w_tau + tau_theta / I_yy;
dot_r = (I_xx - I_yy) / I_zz * q * p + tau_psi / I_zz;

end
